simulink model "Valve"  (R2024b)
settings: Solver=VariableStepAuto  StartTime=0.0  StopTime=10.0  RelTol=1e-3
settings Model: Creator=jackson  LastModifiedBy=jackson

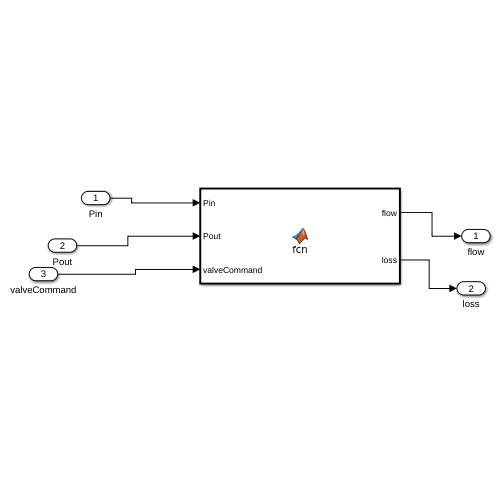
[thumbnail: Simulink's stored preview of the top-level diagram]
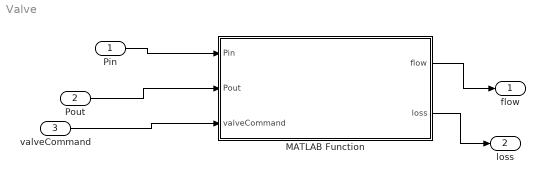
== system Valve ==
  Pin : Inport
  Pout : Inport  Port=2
  valveCommand : Inport  Port=3
  MATLAB Function : MATLAB Function  TreatAsAtomicUnit=on
  flow : Outport
  loss : Outport  Port=2
  wires:
  Pin/1 -> MATLAB Function/1(Pin)
  Pout/1 -> MATLAB Function/2(Pout)
  valveCommand/1 -> MATLAB Function/3(valveCommand)
  MATLAB Function/1(flow) -> flow/1
  MATLAB Function/2(loss) -> loss/1

== matlab function Valve/MATLAB Function ==
  data: Pin input; flow output; Pout input; valveCommand input; params parameter; loss output
function [flow,loss] = fcn(Pin,Pout,valveCommand,params)

flow = valveCommand*params.valveConstant*sqrt(abs(Pout-Pin))*sign(Pout-Pin);
loss = (Pout-Pin)*flow;
